simulink model "SimunlikReference"  (R2021b)
settings: Solver=VariableStepAuto  StartTime=0.0  StopTime=2048*15/fs  RelTol=1e-3
InitFcn:
  | f = 12.288e6;
  | fs = 153.6e6;
  | N = 2048;
  | n = 0:N-1;
  | Hamming = 0.54 + 0.46 * cos(2*pi*n/N);
  | Hanning = 0.5 * (1 + cos(2*pi*n/N));
  | Norm_Ham = sum(Hamming);
  | Norm_Han = sum(Hanning);
undefined symbols (not defined in the file): AXI4, Lite
libraries: hdlBasic x7, dspxfrm3 x2, dspsigops x2, hdlsllib x1, vmcUtilities x1
settings Model: Creator=yxb20126  LastModifiedBy=yxb20126

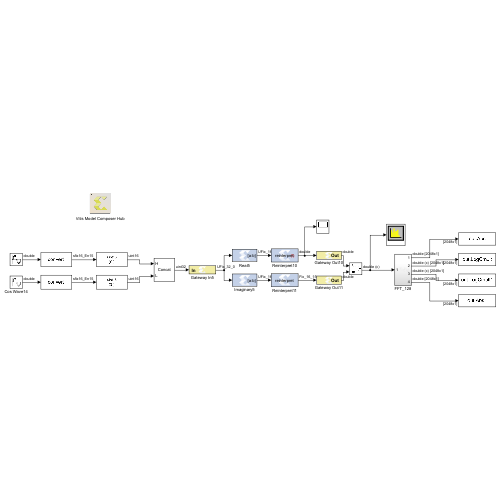
[thumbnail: Simulink's stored preview of the top-level diagram]
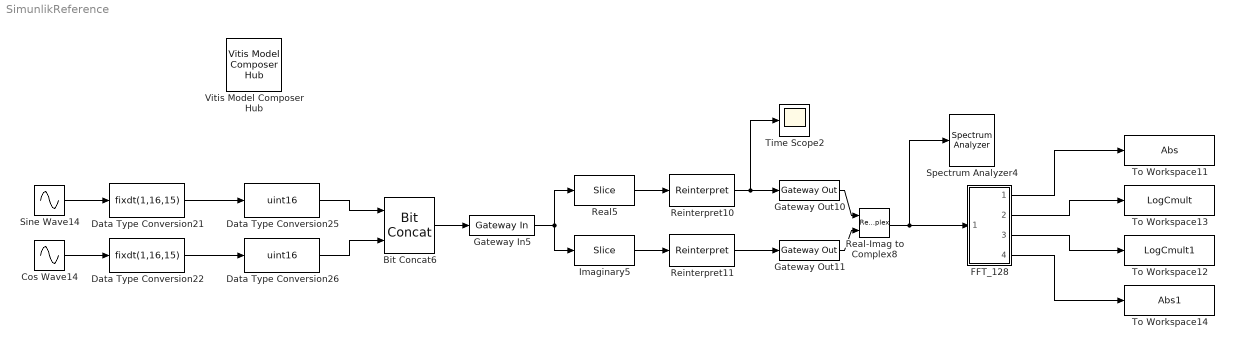
== system SimunlikReference ==
  Bit Concat6 : hdlsllib/Logic and Bit Operations/Bit Concat  numInputs=2
  Cos Wave14 : Sin  Frequency=f*2*pi  Phase=pi/2  SampleTime=1/fs
  Data Type Conversion21 : DataTypeConversion  OutDataTypeStr=fixdt(1,16,15)  SaturateOnIntegerOverflow=on
  Data Type Conversion22 : DataTypeConversion  OutDataTypeStr=fixdt(1,16,15)  SaturateOnIntegerOverflow=on
  Data Type Conversion25 : DataTypeConversion  OutDataTypeStr=uint16  ConvertRealWorld=Stored Integer (SI)
  Data Type Conversion26 : DataTypeConversion  OutDataTypeStr=uint16  ConvertRealWorld=Stored Integer (SI)
  FFT_128 : Subsystem
  Gateway In5 : hdlBasic/Gateway In  gui_display_data_type=Fixed-point  arith_type=Unsigned  n_bits=32  bin_pt=0  preci_type=Single  exp_width=8  frac_width=24  rows=1  columns=1  quantization=Truncate  overflow=Wrap  period=1/fs  UseAsADC=off  ADCChannel='1'  interface=AXI4-Lite  automatic_assignment=on  address_offset=hex2dec('00')  intf_name=''  intf_description=''  default_value=0  timing_constraint=None  locs_specified=off  LOCs={}  io_standard={}  inherit_from_input=off  hdl_port=on  XmcBlockStatus=1  maskContainerNames=group4  block_type=gatewayin  block_config=sysgen:gateway_in_config  block_width_w=590  block_height_w=620  block_width=640  block_height=850
  Gateway Out10 : hdlBasic/Gateway Out  inherit_from_input=off  hdl_port=on  rows=1  columns=1  UseAsDAC=off  DACChannel='1'  interface=AXI4-Lite  automatic_assignment=on  address_offset=hex2dec('00')  intf_name=''  intf_description=''  timing_constraint=None  locs_specified=off  LOCs={}  io_standard={}  XmcBlockStatus=1  maskContainerNames=group4  block_type=gatewayout  block_config=sysgen:gateway_out_config  block_width_w=590  block_height_w=620  block_width=620  block_height=750
  Gateway Out11 : hdlBasic/Gateway Out  inherit_from_input=off  hdl_port=on  rows=1  columns=1  UseAsDAC=off  DACChannel='1'  interface=AXI4-Lite  automatic_assignment=on  address_offset=hex2dec('00')  intf_name=''  intf_description=''  timing_constraint=None  locs_specified=off  LOCs={}  io_standard={}  XmcBlockStatus=1  maskContainerNames=group4  block_type=gatewayout  block_config=sysgen:gateway_out_config  block_width_w=590  block_height_w=620  block_width=620  block_height=750
  Imaginary5 : hdlBasic/Slice  nbits=16  boolean_output=off  mode=Two Bit Locations  bit1=31  base1=LSB of Input  bit0=16  base0=LSB of Input  XmcBlockStatus=1  maskContainerNames=group1  block_type=slice  block_config=sysgen:Slice_config
  Real-Imag to Complex8 : RealImagToComplex
  Real5 : hdlBasic/Slice  nbits=16  boolean_output=off  mode=Two Bit Locations  bit1=15  base1=LSB of Input  bit0=0  base0=LSB of Input  XmcBlockStatus=1  maskContainerNames=group1  block_type=slice  block_config=sysgen:Slice_config
  Reinterpret10 : hdlBasic/Reinterpret  force_arith_type=on  arith_type="Signed  (2's comp)"  force_bin_pt=on  bin_pt=15  XmcBlockStatus=1  maskContainerNames=group1  block_type=reinterpret  block_config=sysgen:Reinterpret_config
  Reinterpret11 : hdlBasic/Reinterpret  force_arith_type=on  arith_type="Signed  (2's comp)"  force_bin_pt=on  bin_pt=15  XmcBlockStatus=1  maskContainerNames=group1  block_type=reinterpret  block_config=sysgen:Reinterpret_config
  Sine Wave14 : Sin  Frequency=f*2*pi  SampleTime=1/fs
  Spectrum Analyzer4 : SpectrumAnalyzer
  Time Scope2 : Scope
  To Workspace11 : ToWorkspace  VariableName=Abs  SampleTime=-1
      settings: Save2DSignal=2-D array (concatenate along first dimension)
  To Workspace12 : ToWorkspace  VariableName=LogCmult1  SampleTime=-1
      settings: Save2DSignal=2-D array (concatenate along first dimension)
  To Workspace13 : ToWorkspace  VariableName=LogCmult  SampleTime=-1
      settings: Save2DSignal=2-D array (concatenate along first dimension)
  To Workspace14 : ToWorkspace  VariableName=Abs1  SampleTime=-1
      settings: Save2DSignal=2-D array (concatenate along first dimension)
  Vitis Model Composer Hub : vmcUtilities/Vitis Model Composer Hub  Tag=genX  CodeGeneration=off  SubsystemName=<enter or select subsystem name>  TargetDirectory=./code  ExportType=HLS C++ code  IpVendor=xilinx.com  IpLibrary=hls  IpVersion=1.0  IpHWLanguage=Verilog  AieCompilerOptions={}  CreateTestbench=off  TestbenchStackSize=10  RunAieSim=off  AieSimTimeout=50000  RunAieSimProfiling=off  LaunchVitisAnalyzer=off  PlotOutput=off  RunX86Sim=off  X86SimTimeout=10  GenHwImage=off  PlatformType=Not Specified  HwSystemType=Baremetal  HwValidationTarget=hw  ProjDevice=xczu48dr-ffvg1517-2-e  ProjDevicePart=xczu48dr-ffvg1517-2-e  SamplePeriod=-1  ClockFrequency=200  DataPathParallelism=1  xilinxfamily=zynquplusRFSOC  part=xczu48dr  speed=-2-e  package=ffvg1517  directory=./netlist  testbench=off  incr_netlist=off  synthesis_tool=Vivado  clock_wrapper=Clock Enables  dbl_ovrd=According to Block Masks  dcm_input_clock_period=10  sysclk_period=(1/fs)*10e9  simulink_period=1/fs  eval_field=0
  wires:
  Reinterpret10/1 -> Time Scope2/1, Gateway Out10/1
  Bit Concat6/1 -> Gateway In5/1
  Gateway Out11/1 -> Real-Imag to Complex8/2
  Imaginary5/1 -> Reinterpret11/1
  Real5/1 -> Reinterpret10/1
  Gateway In5/1 -> Imaginary5/1, Real5/1
  Reinterpret11/1 -> Gateway Out11/1
  Gateway Out10/1 -> Real-Imag to Complex8/1
  FFT_128/1(Out1) -> To Workspace11/1
  FFT_128/2(Out2) -> To Workspace13/1
  FFT_128/3(Out3) -> To Workspace12/1
  FFT_128/4(Out4) -> To Workspace14/1
  Data Type Conversion22/1 -> Data Type Conversion26/1
  Sine Wave14/1 -> Data Type Conversion21/1
  Cos Wave14/1 -> Data Type Conversion22/1
  Data Type Conversion26/1 -> Bit Concat6/2
  Data Type Conversion25/1 -> Bit Concat6/1
  Data Type Conversion21/1 -> Data Type Conversion25/1
  Real-Imag to Complex8/1 -> FFT_128/1(In1), Spectrum Analyzer4/1

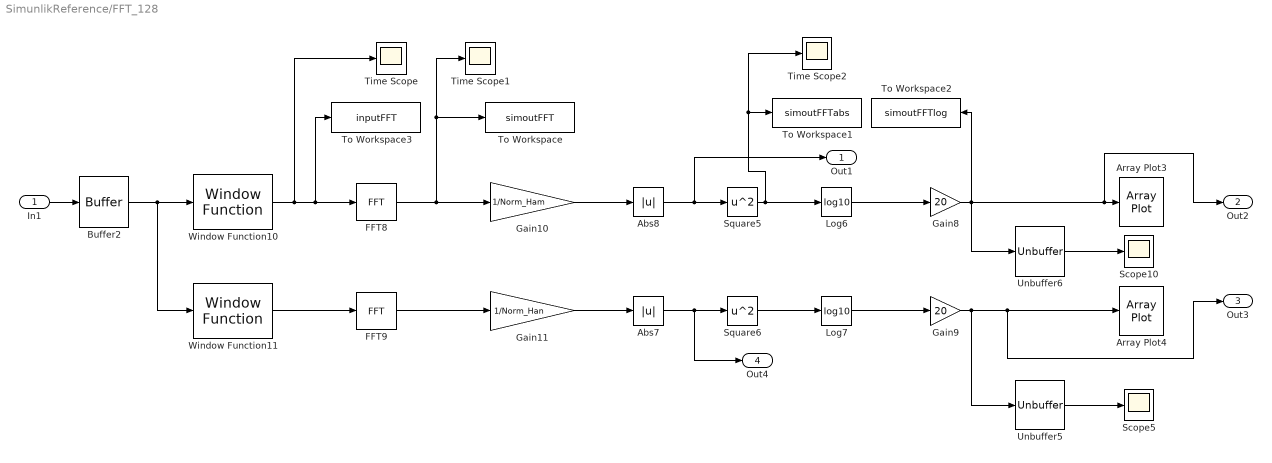
== system SimunlikReference/FFT_128 ==
  In1 : Inport
  Abs7 : Abs
  Abs8 : Abs
  Array Plot3 : ArrayPlot  WindowPosition=[827.000000,398.000000,581.000000,481.000000,]  YLimits=[-59.68956955456875,167.07325575587276]  ShowLegend=on
  Array Plot4 : ArrayPlot  WindowPosition=[214.000000,393.000000,581.000000,481.000000,]  YLimits=[-59.68956955456875,167.07325575587276]  ShowLegend=on
  Buffer2 : Buffer  N=N  OutputFrames=off
  FFT8 : dspxfrm3/FFT  FFTImplementation=Auto  CompMethod=Table lookup  TableOpt=NEW  TableOptActive=Speed  BitRevOrder=off  Normalize=off  InheritFFTLength=off  FFTLength=N  WrapInput=off  roundingMode=Floor  overflowMode=off  firstCoeffDataTypeStr=Inherit: Same word length as input  firstCoeffLastDataTypeStr=Inherit: Same word length as input  outputMin=[]  outputMax=[]
  FFT9 : dspxfrm3/FFT  FFTImplementation=Auto  CompMethod=Table lookup  TableOpt=NEW  TableOptActive=Speed  BitRevOrder=off  Normalize=off  InheritFFTLength=off  FFTLength=N  WrapInput=off  roundingMode=Floor  overflowMode=off  firstCoeffDataTypeStr=Inherit: Same word length as input  firstCoeffLastDataTypeStr=Inherit: Same word length as input  outputMin=[]  outputMax=[]
  Gain10 : Gain  Gain=1/Norm_Ham
  Gain11 : Gain  Gain=1/Norm_Han
  Gain8 : Gain  Gain=20
  Gain9 : Gain  Gain=20
  Log6 : Math  Operator=log10  OutputSignalType=complex  SaturateOnIntegerOverflow=on
  Log7 : Math  Operator=log10  OutputSignalType=complex  SaturateOnIntegerOverflow=on
  Scope10 : Scope
  Scope5 : Scope
  Square5 : Math  Operator=square  SaturateOnIntegerOverflow=on
  Square6 : Math  Operator=square  SaturateOnIntegerOverflow=on
  Time Scope : Scope
  Time Scope1 : Scope
  Time Scope2 : Scope
  To Workspace : ToWorkspace  VariableName=simoutFFT  SampleTime=-1
      settings: Save2DSignal=2-D array (concatenate along first dimension)
  To Workspace1 : ToWorkspace  VariableName=simoutFFTabs  SampleTime=-1
      settings: Save2DSignal=2-D array (concatenate along first dimension)
  To Workspace2 : ToWorkspace  VariableName=simoutFFTlog  SampleTime=-1
      settings: Save2DSignal=2-D array (concatenate along first dimension)
  To Workspace3 : ToWorkspace  VariableName=inputFFT  SampleTime=-1
      settings: Save2DSignal=2-D array (concatenate along first dimension)
  Unbuffer5 : Unbuffer
  Unbuffer6 : Unbuffer
  Window Function10 : dspsigops/Window Function  winmode=Apply window to input  wintype=Hamming  sampmode=Continuous  samptime=1  N=64  Rs=50  beta=10  winsamp=Symmetric  UserWindow=hamming  OptParams=off  UserParams={'symmetric'}  dataType=double  isSigned=on  wordLen=16  udDataType=sfix(16)  fracBitsMode=Best precision  numFracBits=15  roundingMode=Floor  overflowMode=on  numSidelobes=4  sidelobeLevel=-30
      settings: SourceProductBaseCode=DS
  Window Function11 : dspsigops/Window Function  winmode=Apply window to input  wintype=Hann  sampmode=Continuous  samptime=1  N=64  Rs=50  beta=10  winsamp=Symmetric  UserWindow=hamming  OptParams=off  UserParams={'symmetric'}  dataType=double  isSigned=on  wordLen=16  udDataType=sfix(16)  fracBitsMode=Best precision  numFracBits=15  roundingMode=Floor  overflowMode=on  numSidelobes=4  sidelobeLevel=-30
      settings: SourceProductBaseCode=DS
  Out1 : Outport
  Out2 : Outport  Port=2
  Out3 : Outport  Port=3
  Out4 : Outport  Port=4
  wires:
  FFT8/1 -> Time Scope1/1, To Workspace/1, Gain10/1
  Unbuffer6/1 -> Scope10/1
  Log6/1 -> Gain8/1
  Gain8/1 -> To Workspace2/1, Out2/1, Array Plot3/1, Unbuffer6/1
  Square5/1 -> Time Scope2/1, To Workspace1/1, Log6/1
  Gain9/1 -> Out3/1, Array Plot4/1, Unbuffer5/1
  Buffer2/1 -> Window Function11/1, Window Function10/1
  Abs8/1 -> Out1/1, Square5/1
  Window Function11/1 -> FFT9/1
  Log7/1 -> Gain9/1
  Square6/1 -> Log7/1
  Window Function10/1 -> Time Scope/1, To Workspace3/1, FFT8/1
  Unbuffer5/1 -> Scope5/1
  In1/1 -> Buffer2/1
  Abs7/1 -> Out4/1, Square6/1
  Gain10/1 -> Abs8/1
  Gain11/1 -> Abs7/1
  FFT9/1 -> Gain11/1
